simulink model "test_sim"  (R2023b)
settings: Solver=VariableStepAuto  StartTime=0.0  StopTime=10  RelTol=1e-3
values from neighbouring files (symbols this model uses):
  A_ob = A - L_kf*C    [LQ_KF_version1.m]    (also in LQ_KF_version2.m; LQ_Luenberger.m; PP_Luenberger.m = A - L*C; prova1.m = A - L*C)
  B_ob = [ B - L_kf*D, L_kf]    [LQ_KF_version1.m]    (also in LQ_KF_version2.m; LQ_Luenberger.m; PP_Luenberger.m = [ B, L]; prova1.m = [ B, L])
  C_ob = eye(n)    [LQ_KF_version1.m]    (also in LQ_KF_version2.m; LQ_Luenberger.m; PP_Luenberger.m; prova1.m)
  D_ob = zeros(n, m+p)    [LQ_KF_version1.m]    (also in LQ_KF_version2.m; LQ_Luenberger.m; PP_Luenberger.m; prova1.m)
undefined symbols (not defined in the file or in its folder): x1_eq0, x2_eq0
libraries: simulink x3
settings Model: Creator=lollo  LastModifiedBy=lollo

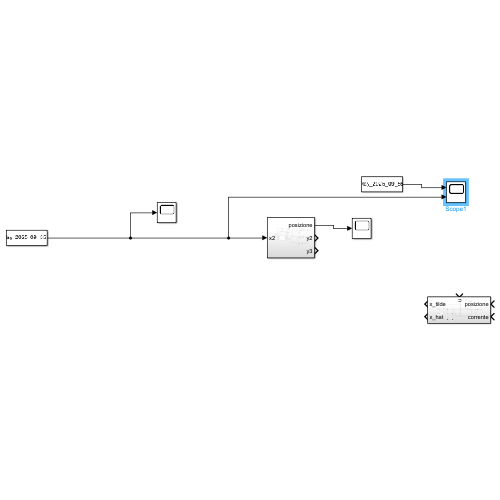
[thumbnail: Simulink's stored preview of the top-level diagram]
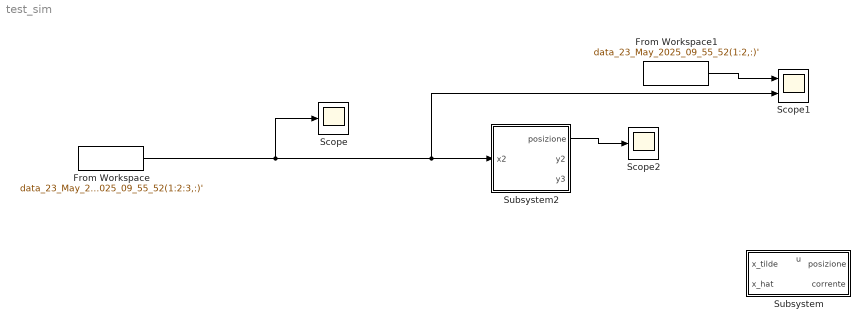
== system test_sim ==
  From Workspace : FromWorkspace  VariableName=data_23_May_2025_09_55_52(1:2:3,:)'
  From Workspace1 : FromWorkspace  VariableName=data_23_May_2025_09_55_52(1:2,:)'
  Scope : Scope
  Scope1 : Scope  NumInputPorts=2
  Scope2 : Scope
  Subsystem : Subsystem
      settings: PortSchema="{\"entries\":[{\"content\":{\"sides\":[{\"content\":{\"connectorIds\":[\"In1\",\"In2\"]},\"type\":\"ConnectorPlacement.EquallySpacedRectSide\",\"uuid\":\"698df1f3-7755-43c0-a5fb-5bdaf8e9b8ef\"},{\"content\":{\"connectorIds\":[\"Out1\",\"Out2\"],\"side\":\"RIGHT\"},\"type\":\"ConnectorPlacement.EquallySpacedRectSide\",\"uuid\":\"f0019f40-b27c-431f-9c37-04fd54da4bcb\"},{\"content\":{\"connectorIds\":[\"In3\"],\"side\":\"TOP\"},\"type\":\"ConnectorPlacement.EquallySpacedRectSide\",\"uuid\":\"7983fe5a-f7de-4e42-be2b-50e780fdde63\"}]},\"type\":\"ConnectorPlacement.EquallySpacedConnector\",\"uuid\":\"65d76084-d1f3-463d-b10f-a9e5fd5bbc83\"}],\"packageUris\":[\"http://schema.mathworks.com/mf0/Connector/R2020b\"],\"version\":\"1.0\"}"
  Subsystem2 : Subsystem
  wires:
  From Workspace1/1 -> Scope1/1
  From Workspace/1 -> Scope/1, Scope1/2, Subsystem2/1(x2)
  Subsystem2/1(posizione) -> Scope2/1

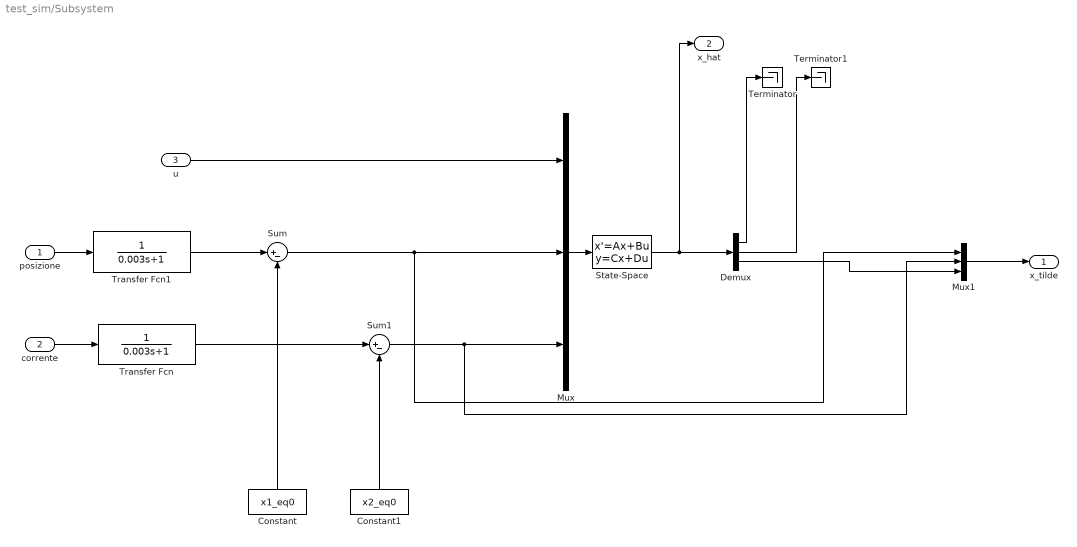
== system test_sim/Subsystem ==
  posizione : Inport
  corrente : Inport  Port=2
  u : Inport  Port=3
  Constant : Constant  Value=x1_eq0
  Constant1 : Constant  Value=x2_eq0
  Demux : Demux  Outputs=3
  Mux : Mux  Inputs=3
  Mux1 : Mux  Inputs=3
  State-Space : StateSpace  A=A_ob  B=B_ob  C=C_ob  D=D_ob  InitialCondition=[-x1_eq0, -x2_eq0, 0]  ParameterTunability=Unconstrained
  Sum : Sum  Inputs=|+-
  Sum1 : Sum  Inputs=|+-
  Terminator : Terminator
  Terminator1 : Terminator
  Transfer Fcn : TransferFcn  Denominator=[0.003 1]
  Transfer Fcn1 : TransferFcn  Denominator=[0.003 1]
  x_tilde : Outport
  x_hat : Outport  Port=2
  wires:
  posizione/1 -> Transfer Fcn1/1
  Constant/1 -> Sum/2
  Constant1/1 -> Sum1/2
  corrente/1 -> Transfer Fcn/1
  u/1 -> Mux/1
  Sum/1 -> Mux1/1, Mux/2
  Sum1/1 -> Mux1/2, Mux/3
  Mux/1 -> State-Space/1
  Mux1/1 -> x_tilde/1
  State-Space/1 -> x_hat/1, Demux/1
  Demux/1 -> Terminator/1
  Demux/2 -> Terminator1/1
  Demux/3 -> Mux1/3
  Transfer Fcn/1 -> Sum1/1
  Transfer Fcn1/1 -> Sum/1

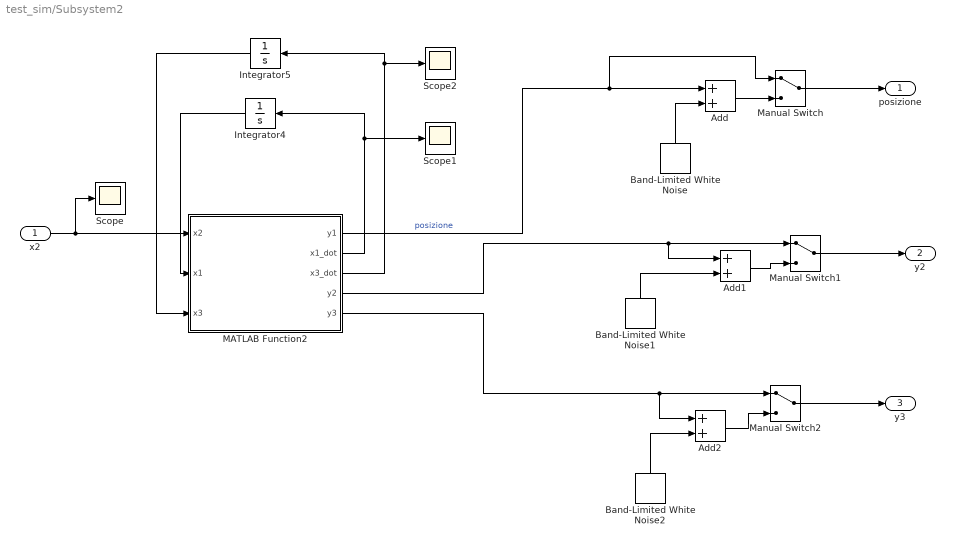
== system test_sim/Subsystem2 ==
  x2 : Inport
  Add : Sum
  Add1 : Sum
  Add2 : Sum
  Band-Limited White Noise : simulink/Sources/Band-Limited White Noise  Cov=[8.9934e-8*0.002]  Ts=0.002  seed=[23341]
  Band-Limited White Noise1 : simulink/Sources/Band-Limited White Noise  Cov=[8.9934e-8*0.002]  Ts=0.002  seed=[23341]
  Band-Limited White Noise2 : simulink/Sources/Band-Limited White Noise  Cov=[8.9934e-8*0.002]  Ts=0.002  seed=[23341]
  Integrator4 : Integrator
  Integrator5 : Integrator
  MATLAB Function2 : MATLAB Function  TreatAsAtomicUnit=on
  Manual Switch : ManualSwitch
  Manual Switch1 : ManualSwitch
  Manual Switch2 : ManualSwitch
  Scope : Scope
  Scope1 : Scope
  Scope2 : Scope
  posizione : Outport
  y2 : Outport  Port=2
  y3 : Outport  Port=3
  wires:
  Integrator5/1 -> MATLAB Function2/3(x3)
  MATLAB Function2/2(x1_dot) -> Scope1/1, Integrator4/1
  MATLAB Function2/3(x3_dot) -> Scope2/1, Integrator5/1
  Integrator4/1 -> MATLAB Function2/2(x1)
  x2/1 -> Scope/1, MATLAB Function2/1(x2)
  Manual Switch/1 -> posizione/1
  Manual Switch1/1 -> y2/1
  Manual Switch2/1 -> y3/1
  Add/1 -> Manual Switch/2
  Band-Limited White Noise/1 -> Add/2
  Add1/1 -> Manual Switch1/2
  Band-Limited White Noise1/1 -> Add1/2
  Add2/1 -> Manual Switch2/2
  Band-Limited White Noise2/1 -> Add2/2
  MATLAB Function2/1(y1) -> Manual Switch/1, Add/1  "posizione"
  MATLAB Function2/4(y2) -> Add1/1, Manual Switch1/1
  MATLAB Function2/5(y3) -> Add2/1, Manual Switch2/1

== matlab function test_sim/Subsystem2/MATLAB Function2 ==
  data: y1 output; x2 input; x1_dot output; x1 input; x3 input; x3_dot output; y2 output; y3 output
function [y1,x1_dot, x3_dot, y2, y3] = fcn(x2, x1, x3)
    m = 0.0657;
    g = 9.81;
    k_mag = 2.4405e-05;
    
    Rtot = 9.7585;
    Lc = 0.3708;
    y0 = 0.012;
    
    x1_dot = x3;
    x3_dot = (k_mag/m)*(x2/(y0-x1))^2 - g;

    if x1 <= 0 && x3_dot < 0
        x1 = 0;
        x3 = 0;
        x3_dot = 0;
    end
y1 = x1;
y2 = x2;
y3 = x3;
